simulink model "TP1_2"  (R2022a)
settings: Solver=VariableStepAuto  StartTime=0.0  StopTime=10.0  RelTol=1e-3
settings Model: Creator=acanon  LastModifiedBy=acanon

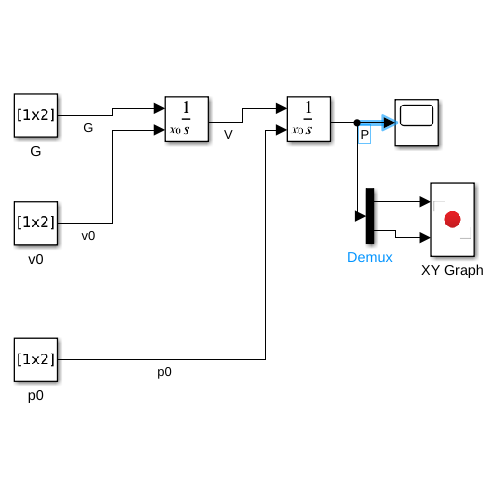
[thumbnail: Simulink's stored preview of the top-level diagram]
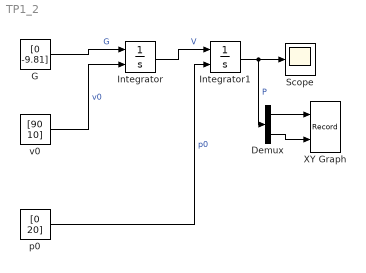
== system TP1_2 ==
  Demux : Demux  Outputs=2
  G : Constant  Value=[0 -9.81]
  Integrator : Integrator  InitialConditionSource=external
  Integrator1 : Integrator  InitialConditionSource=external
  Scope : Scope
  XY Graph : Record  FileSettingsInternal="{\"entries\":[{\"content\":{\"excelSettings\":{\"content\":{},\"type\":\"Streamout.ExcelSettings\"}},\"type\":\"Streamout.FileSettingStorage\",\"uuid\":\"c4c6623e-7de9-46e1-a7a8-2e545214fc93\"}],\"packageUris\":[\"http://schema.mathworks.com/mf0/streamout_blocks/R2020a\"],\"version\":\"1.0\"}"  Layout=[1 1]  SignalsInternal="{\"entries\":[{\"content\":{\"signals\":[{\"content\":{\"blockPath\":[\"untitled/XY Graph\"],\"channel\":[],\"dimensions\":[1],\"domain\":\"untitled/XY Graph\",\"lineColor\":\"#a2142f\",\"plots\":[1],\"port\":1,\"sid\":[\"\"],\"signalID\":30,\"signalName\":\"Demux:1\"},\"type\":\"RecordBlkView.Signal\",\"uuid\":\"791e067e-83fc-41a3-a8a2-178d5d401975\"},{\"content\":{\"blockPath\":[\"untitled/XY Graph\"],\"channel\":[],\"dimensions\":[1],\"domain\":\"untitled/XY Graph\",\"lineColor\":\"#139fff\",\"plots\":[1],\"port\":2,\"sid\":[\"\"],\"signalID\":34,\"signalName\":\"Demux:2\"},\"type\":\"RecordBlkView.Signal\",\"uuid\":\"04911b83-3768-459b-95ce-24f86e0a8442\"}]},\"type\":\"RecordBlkView.InputSignals\",\"uuid\":\"68908274-827a-4599-bf5b-9f8dab8a4317\"}],\"packageUris\":[\"http://schema.mathworks.com/mf0/streamout_blocks/R2020a\"],\"version\":\"1.0\"}"  VisualizationBindings="{\"xyplotplugin\":{\"info\":[{\"series\":[{\"bindingParametersList\":[{\"parameter\":\"X-Axis\",\"signalID\":30,\"signalName\":\"Demux:1\"},{\"parameter\":\"Y-Axis\",\"signalID\":34,\"signalName\":\"Demux:2\"}],\"seriesID\":44633}],\"subplotID\":1}]}}"  CompatibilityTag=XY
  p0 : Constant  Value=[0 20]
  v0 : Constant  Value=[90 10]
  wires:
  G/1 -> Integrator/1  "G"
  Integrator/1 -> Integrator1/1  "V"
  v0/1 -> Integrator/2  "v0"
  p0/1 -> Integrator1/2  "p0"
  Integrator1/1 -> Demux/1, Scope/1  "P"
  Demux/1 -> XY Graph/1
  Demux/2 -> XY Graph/2
